simulink model "SingleModuleWithPresetValue"  (R2016a)
settings: Solver=VariableStepAuto  StartTime=0.0  StopTime=0.4  RelTol=1e-3
undefined symbols (not defined in the file): freq
libraries: powerlib x6, powerlib_meascontrol x6, fl_lib x3, nesl_utility x3, dspstat3 x1
settings Model: Creator=ugurm  LastModifiedBy=kkfrk

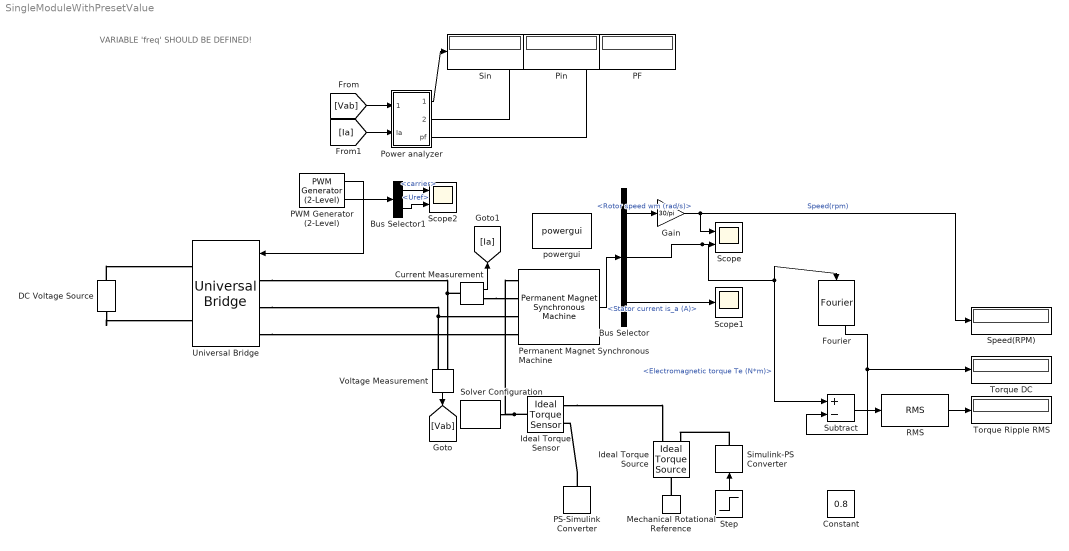
== system SingleModuleWithPresetValue ==
  note: VARIABLE 'freq' SHOULD BE DEFINED!
  Bus Selector : BusSelector  OutputSignals=Rotor speed wm (rad/s),Electromagnetic torque Te (N*m),Stator current is_a (A)
  Bus Selector1 : BusSelector  OutputSignals=carrier,Uref
  Constant : Constant  Value=0.8
  Current Measurement : powerlib/Measurements/Current Measurement  PhasorSimulation=off  OutputType=Complex  PSBequivalent=0
  DC Voltage Source : powerlib/Electrical Sources/DC Voltage Source  Amplitude=300  Measurements=None
  Fourier : powerlib_meascontrol/Measurements/Fourier  Freq=freq  n=0  InInit=[0, 0]  Ts=0
  Gain : Gain  Gain=30/pi
  Ideal Torque Sensor : fl_lib/Mechanical/Mechanical Sensors/Ideal Torque Sensor
  Ideal Torque Source : fl_lib/Mechanical/Mechanical Sources/Ideal Torque Source
  Mechanical Rotational Reference : fl_lib/Mechanical/Rotational Elements/Mechanical Rotational Reference
  PF : Display
  PS-Simulink Converter : nesl_utility/PS-Simulink Converter  PhysicalDomain=network_engine_domain  SubClassName=ps_output  LeftPortType=input  RightPortType=output  PseudoPeriodic=off  Frequencies=[]  Unit=1  AffineConversion=off
  PWM Generator (2-Level) : powerlib_meascontrol/Pulse & Signal Generators/PWM Generator (2-Level)  ModulatorType=Three-phase bridge (6 pulses)  ModulatorMode=Unsynchronized  Fc=27*freq  Pc=90  nF=27  MinMax="[ -1  1 ]"  SamplingTechnique=Natural  ModulatingSignals=on  m=0.8  Freq=freq  Phase=0  Ts=0  ShowCarrierOutport=on
  Permanent Magnet Synchronous Machine : powerlib/Machines/Permanent Magnet Synchronous Machine  NbPhases=3  FluxDistribution=Sinusoidal  RotorType=Round  MechanicalLoad=Mechanical rotational port  PresetModel="01:  0.8 Nm 300 Vdc 3000 RPM - 0.8 Nm"  ShowDetailedParameters=on  MeasurementBus=off  Resistance=18.7  Inductance=8.5e-3  dqInductances=[0.0009642 0.001066]  La=0.02682  MachineConstant=Flux linkage established by magnets (V.s)  Flux=0.1717  VoltageCst=67.038  TorqueCst=0.5544  Flat=120  Mechanical=[2.26e-05 1.349e-05 2 0]  PolePairs=2  InitialConditions=[0,0, 0,0]  InitialConditions5ph=[0 0 0 0 0 0]  TsPowergui=0  TsBlock=-1  RefAngle=90 degrees behind phase A axis (modified Park)
  Pin : Display
  Power analyzer : Subsystem  RequirementInfo="{}  %GIDa_8630ca45_a338_4afd_a5f7_96069bb0fd47"
  RMS : dspstat3/RMS  run=off  reset_popup=None  InputProcessing=Columns as channels (frame based)  directionMode=Each column  dimension=1
  Scope : Scope  NumInputPorts=2
  Scope1 : Scope
  Scope2 : Scope  NumInputPorts=2
  Simulink-PS Converter : nesl_utility/Simulink-PS Converter  PhysicalDomain=network_engine_domain  SubClassName=ps_input  LeftPortType=input  RightPortType=output  PseudoPeriodic=off  Frequencies=[]  NoiseDistribution=none  NoiseParameters=[]  Unit=1  AffineConversion=off  InputFiltering=off  SimscapeFilterOrder=1  InputFilterTimeConstant=0.001  UdotUserProvided=1
  Sin : Display
  Solver Configuration : nesl_utility/Solver Configuration  PhysicalDomain=network_engine_domain  SubClassName=solver  LeftPortType=input  RightPortType=generic  Accelerate=off  Tones=[]  Harmonics=[]  SimulateNoise=off  Profile=off  UseLocalSampling=off  EnableSwitchedLinearOptims=on  FrequencyDomain=off  UseCCode=off  RelTol=0.001  AbsTol=1e-06  MinStep=1e-09  ToWorkspace=off  RevertToSquareIcSolve=off  NumHomotopyIterations=100  PhasorMode=off  PhasorModeNumHarmonics=1  OverrideAbsTol=off  DoDC=off  ResidualTolerance=1e-09  UseLocalSolver=on  LocalSolverChoice=NE_BACKWARD_EULER_ADVANCER  LocalSolverSampleTime=1e-6  DoFixedCost=on  MaxNonlinIter=3  MaxModeIter=2  LinearAlgebra=Sparse  DelaysMemoryBudget=1024  AutomaticFiltering=on  FilteringTimeConstant=0.001
  Speed(RPM) : Display
  Step : Step  Time=0.2  After=0.5  SampleTime=0
  Subtract : Sum  Inputs=+-
  Torque DC : Display
  Torque Ripple RMS : Display
  Universal Bridge : powerlib/Power Electronics/Universal Bridge  Arms=3  SnubberResistance=1e5  SnubberCapacitance=inf  Device=IGBT / Diodes  Ron=1e-3  Lon=0  ForwardVoltages="[  0  0  ]"  ForwardVoltage=0  GTOparameters=[ 10e-6 , 20e-6 ]  IGBTparameters=[ 1e-6 , 2e-6 ]  Measurements=None  Measurements_2=None  converterType=Rectifier
  Voltage Measurement : powerlib/Measurements/Voltage Measurement  PhasorSimulation=off  OutputType=Complex  PSBequivalent=0
  powergui : powerlib/powergui  Priority=1  SimulationMode=Discrete  SolverType=Tustin/Backward Euler (TBE)  SampleTime=1e-6  frequency=60  SPID=off  DisableSnubberDevices=off  DisableRonSwitches=off  DisableVfSwitches=off  SwTol=0  DisplayEquations=off  Interpol=off  ExternalGateDelay=off  methode=off  Ts=10  FunctionMessages=off  echomessages=off  HookPort=off  EnableUseOfTLC=off  x0status=blocks  frequencyindice=0  Pbase=100e6  ErrMax=1e-4  Iterations=50  UnitsV=kV  UnitsW=MW  buscounter=0  RestoreLinks=warning  ResistiveCurrentMeasurement=off  Frange=[0:2:500]  Ylog=off  Xlog=on  ShowGrid=off  save=off  variable=ZData  structure=0  ZoomFFT=off  StartTime=0.0  cycles=1  DisplayStyle=1  fundamental=60  FreqAxis=off  MaxFrequency=1000  frequencyindicesteady=1  RmsSteady=1  display=off
  wires:
  Permanent Magnet Synchronous Machine/1 -> Bus Selector/1
  Bus Selector/1 -> Gain/1  "<Rotor speed wm (rad/s)>"
  Bus Selector/2 -> Subtract/1, Fourier/1, Scope/2  "<Electromagnetic torque Te (N*m)>"
  Bus Selector/3 -> Scope1/1  "<Stator current is_a (A)>"
  Voltage Measurement/1 -> [Vab]
  [Vab] -> Power analyzer/1(Vab)
  [Ia] -> Power analyzer/2(Ia)
  Current Measurement/1 -> [Ia]
  Power analyzer/1(Sin) -> Sin/1
  Power analyzer/2(Pin) -> Pin/1
  Power analyzer/3(pf) -> PF/1
  PWM Generator (2-Level)/1 -> Universal Bridge/1
  PWM Generator (2-Level)/2 -> Bus Selector1/1
  Bus Selector1/1 -> Scope2/1  "<carrier>"
  Bus Selector1/2 -> Scope2/2  "<Uref>"
  Step/1 -> Simulink-PS Converter/1
  Fourier/1 -> Subtract/2, Torque DC/1
  Subtract/1 -> RMS/1
  RMS/1 -> Torque Ripple RMS/1
  Gain/1 -> Speed(RPM)/1, Scope/1  "Speed(rpm)"
  connections:
  Ideal Torque Sensor/LConn1 -- Permanent Magnet Synchronous Machine/LConn1 -- Solver Configuration/RConn1
  Ideal Torque Sensor/RConn1 -- Ideal Torque Source/RConn2
  Mechanical Rotational Reference/LConn1 -- Ideal Torque Source/LConn1
  Simulink-PS Converter/RConn1 -- Ideal Torque Source/RConn1
  PS-Simulink Converter/LConn1 -- Ideal Torque Sensor/RConn2
  Current Measurement/LConn1 -- Universal Bridge/LConn1 -- Voltage Measurement/LConn1
  Voltage Measurement/LConn2 -- Universal Bridge/LConn2 -- Permanent Magnet Synchronous Machine/LConn3
  Current Measurement/RConn1 -- Permanent Magnet Synchronous Machine/LConn2
  Universal Bridge/LConn3 -- Permanent Magnet Synchronous Machine/LConn4
  DC Voltage Source/LConn1 -- Universal Bridge/RConn2
  DC Voltage Source/RConn1 -- Universal Bridge/RConn1

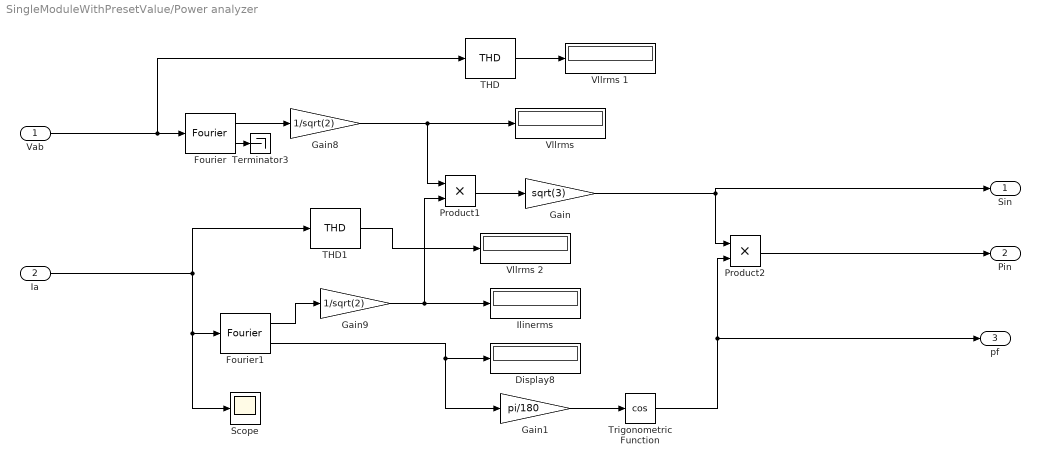
== system SingleModuleWithPresetValue/Power analyzer ==
  Vab : Inport
  Ia : Inport  Port=2
  Display8 : Display
  Fourier : powerlib_meascontrol/Measurements/Fourier  Freq=freq  n=1  InInit=[0, 0]  Ts=0
  Fourier1 : powerlib_meascontrol/Measurements/Fourier  Freq=freq  n=1  InInit=[0, 0]  Ts=0
  Gain : Gain  Gain=sqrt(3)
  Gain1 : Gain  Gain=pi/180
  Gain8 : Gain  Gain=1/sqrt(2)
  Gain9 : Gain  Gain=1/sqrt(2)
  "Ilinerms " : Display
  Product1 : Product
  Product2 : Product
  Scope : Scope
  THD : powerlib_meascontrol/Measurements/THD  Freq=freq  Ts=0
  THD1 : powerlib_meascontrol/Measurements/THD  Freq=freq  Ts=0
  Terminator3 : Terminator
  Trigonometric Function : Trigonometry  Operator=cos
  "Vllrms " : Display
  Vllrms 1 : Display
  Vllrms 2 : Display
  Sin : Outport
  Pin : Outport  Port=2
  pf : Outport  Port=3
  wires:
  Gain8/1 -> Product1/1, "Vllrms "/1
  Gain9/1 -> "Ilinerms "/1, Product1/2
  Ia/1 -> Scope/1, Fourier1/1, THD1/1
  Fourier1/1 -> Gain9/1
  Vab/1 -> THD/1, Fourier/1
  Fourier/1 -> Gain8/1
  Product1/1 -> Gain/1
  Gain/1 -> Sin/1, Product2/1
  Fourier1/2 -> Gain1/1, Display8/1
  Trigonometric Function/1 -> pf/1, Product2/2
  Gain1/1 -> Trigonometric Function/1
  Product2/1 -> Pin/1
  Fourier/2 -> Terminator3/1
  THD/1 -> Vllrms 1/1
  THD1/1 -> Vllrms 2/1
